simulink model "sfbuilder_euler2dc"  (Simulink 7.6)
settings: Solver=FixedStepDiscrete  StartTime=0.0  StopTime=10.0  FixedStep=0.020  RelTol=1e-3
values from neighbouring files (symbols this model uses):
  D = [-3    0 ... (first row only)    [csfunc.m]    (also in dsfunc.m = [   -0.8141   -2.9334)
settings Model: Creator=The MathWorks Inc.  ExtModeAutoUpdateStatusClock=off
settings DataIOCC: SignalLoggingName=sigsOut
settings OptimizationCC: BooleanDataType=off  InlineInvariantSignals=on
settings DebuggingCC: SaveWithParameterizedLinksMsg=none  SolverPrmCheckMsg=none  MultiTaskDSMMsg=warning  MultiTaskCondExecSysMsg=none
settings HardwareCC: ProdHWDeviceType=Specified
settings RTWCC: IncludeERTFirstTime=on
settings GRTTargetCC: TargetFcnLib=iso_c_tmw.mat

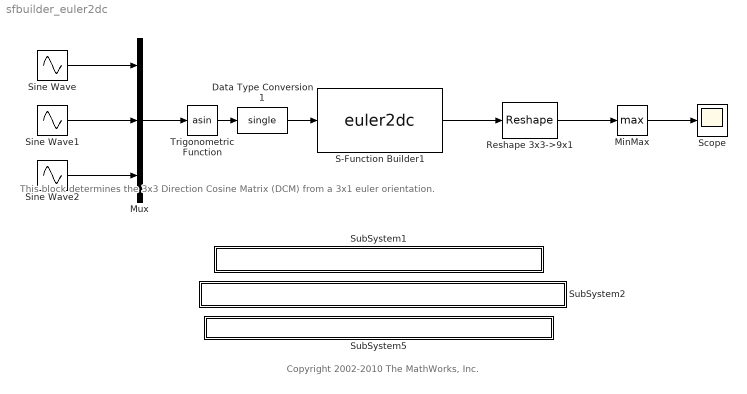
== system sfbuilder_euler2dc ==
  note: This block determines the 3x3 Direction Cosine Matrix (DCM)
      | from a 3x1 euler orientation.
  note: Copyright 2002-2010 The MathWorks, Inc.
  Data Type Conversion1 : DataTypeConversion  OutDataTypeStr=single  SaturateOnIntegerOverflow=on  RndMeth=Zero
  MinMax : MinMax  Function=max  ZeroCross=off  SaturateOnIntegerOverflow=on  InputSameDT=on
  Mux : Mux  Inputs=3
  Reshape 3x3->9x1 : Reshape  OutputDimensionality=Column vector (2-D)  OutputDimensions=[3,3]
  S-Function Builder1 : S-Function  FunctionName=euler2dc  SFunctionModules=euler2dc_wrapper  WizardData=DataTag0  EnableBusSupport=off  mask(S-Function Builder){}
      mask init:
      | val = [[.9  0.75 0.75 1 1 .9 .9 1]',[1 1 0.75 0.75 .9 .9 1 .9]'];
      | sys = get_param(gcb,'FunctionName');
      settings: CopyFcn=set_param(gcb,'LinkStatus','none')  OpenFcn=sfunctionwizard(gcbh)
      mask Display:
      | plot(val(:,1),val(:,2))
      | disp(sys)
      | port_label('input',1,'worke')
      | port_label('output',1,'dircos')
  Scope : Scope
      settings: TimeRange=10  YMin=0.6  YMax=1
  Sine Wave : Sin  SampleTime=0
  Sine Wave1 : Sin  Phase=1  SampleTime=0
  Sine Wave2 : Sin  Phase=2  SampleTime=0
  SubSystem1 : Subsystem  mask{filename=euler2dc.c}
      mask init:
      | x=sfundemo_maskdisp;
      settings: AttributesFormatString=\n  OpenFcn=sfundemo_openfcn
      mask Display: disp(x);
  SubSystem2 : Subsystem  mask{filename=euler2dc_wrapper.c}
      mask init:
      | x=sfundemo_maskdisp;
      settings: AttributesFormatString=\n  OpenFcn=sfundemo_openfcn
      mask Display: disp(x);
  SubSystem5 : Subsystem  mask{filename=euler2dc.tlc}
      mask init:
      | x=sfundemo_maskdisp;
      settings: AttributesFormatString=\n  OpenFcn=sfundemo_openfcn
      mask Display: disp(x);
  Trigonometric Function : Trigonometry  Operator=asin
  wires:
  Sine Wave/1 -> Mux/1
  Sine Wave1/1 -> Mux/2
  Sine Wave2/1 -> Mux/3
  Mux/1 -> Trigonometric Function/1
  Trigonometric Function/1 -> Data Type Conversion1/1
  S-Function Builder1/1 -> Reshape 3x3->9x1/1
  Reshape 3x3->9x1/1 -> MinMax/1
  Data Type Conversion1/1 -> S-Function Builder1/1
  MinMax/1 -> Scope/1

== system sfbuilder_euler2dc/SubSystem1 ==

== system sfbuilder_euler2dc/SubSystem2 ==

== system sfbuilder_euler2dc/SubSystem5 ==
